simulink model "Allgemeine_Schematische"  (Simulink 7.7)
settings: Solver=ode45  StartTime=0.0  StopTime=12  MinStep=0.0001  RelTol=1e-3
undefined symbols (not defined in the file or in its folder): quad
libraries: simulink x4
settings Model: Creator=evgenov  LastModifiedBy=Alexey
settings DebuggingCC: FcnCallInpInsideContextMsg=Enable All

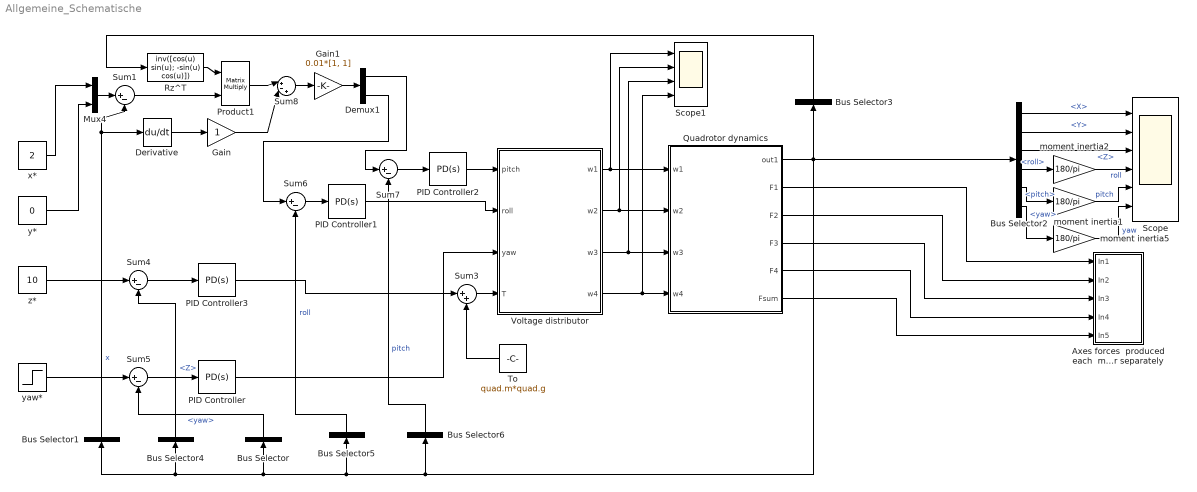
== system Allgemeine_Schematische ==
  Axes forces  produced each  motor separately : Subsystem
  Bus Selector : BusSelector  OutputSignals=yaw
  Bus Selector1 : BusSelector  OutputSignals=X,Y  OutputAsBus=on
  Bus Selector2 : BusSelector  OutputSignals=X,Y,Z,roll,pitch,yaw
  Bus Selector3 : BusSelector  OutputSignals=yaw  OutputAsBus=on
  Bus Selector4 : BusSelector  OutputSignals=Z
  Bus Selector5 : BusSelector  OutputSignals=roll  OutputAsBus=on
  Bus Selector6 : BusSelector  OutputSignals=pitch  OutputAsBus=on
  Demux1 : Demux  Outputs=2
  Derivative : Derivative
  Gain : Gain
  Gain1 : Gain  Gain=0.01*[1, 1]
  Mux4 : Mux  Inputs=2
  PID Controller : simulink/Continuous/PID Controller  SystemSampleTime=-1  Controller=PD  TimeDomain=Continuous-time  SampleTime=1  IntegratorMethod=Forward Euler  FilterMethod=Forward Euler  Form=Parallel  P=1  I=1  D=1  N=100  InitialConditionSource=internal  InitialConditionForIntegrator=0  InitialConditionForFilter=0  ExternalReset=none  LimitOutput=off  UpperSaturationLimit=inf  LowerSaturationLimit=-inf  LinearizeAsGain=off  AntiWindupMode=none  Kb=1  TrackingMode=off  Kt=1  PParamMin=[]  PParamMax=[]  IParamMin=[]  IParamMax=[]  DParamMin=[]  DParamMax=[]  NParamMin=[]  NParamMax=[]  KbParamMin=[]  KbParamMax=[]  KtParamMin=[]  KtParamMax=[]  POutMin=[]  POutMax=[]  IOutMin=[]  IOutMax=[]  DOutMin=[]  DOutMax=[]  NOutMin=[]  NOutMax=[]  KbOutMin=[]  KbOutMax=[]  KtOutMin=[]  KtOutMax=[]  IntegratorOutMin=[]  IntegratorOutMax=[]  FilterOutMin=[]  FilterOutMax=[]  SumOutMin=[]  SumOutMax=[]  SumI1OutMin=[]  SumI1OutMax=[]  SumI2OutMin=[]  SumI2OutMax=[]  SumI3OutMin=[]  SumI3OutMax=[]  SumDOutMin=[]  SumDOutMax=[]  SaturationOutMin=[]  SaturationOutMax=[]  IntegratorContinuousStateAttributes=''  IntegratorStateMustResolveToSignalObject=off  IntegratorRTWStateStorageClass=Auto  FilterContinuousStateAttributes=''  FilterStateMustResolveToSignalObject=off  FilterRTWStateStorageClass=Auto
  PID Controller1 : simulink/Continuous/PID Controller  SystemSampleTime=-1  Controller=PD  TimeDomain=Continuous-time  SampleTime=1  IntegratorMethod=Forward Euler  FilterMethod=Forward Euler  Form=Parallel  P=1  I=0  D=1  N=100  InitialConditionSource=internal  InitialConditionForIntegrator=0  InitialConditionForFilter=0  ExternalReset=none  LimitOutput=off  UpperSaturationLimit=inf  LowerSaturationLimit=-inf  LinearizeAsGain=off  AntiWindupMode=none  Kb=1  TrackingMode=off  Kt=1  PParamMin=[]  PParamMax=[]  IParamMin=[]  IParamMax=[]  DParamMin=[]  DParamMax=[]  NParamMin=[]  NParamMax=[]  KbParamMin=[]  KbParamMax=[]  KtParamMin=[]  KtParamMax=[]  POutMin=[]  POutMax=[]  IOutMin=[]  IOutMax=[]  DOutMin=[]  DOutMax=[]  NOutMin=[]  NOutMax=[]  KbOutMin=[]  KbOutMax=[]  KtOutMin=[]  KtOutMax=[]  IntegratorOutMin=[]  IntegratorOutMax=[]  FilterOutMin=[]  FilterOutMax=[]  SumOutMin=[]  SumOutMax=[]  SumI1OutMin=[]  SumI1OutMax=[]  SumI2OutMin=[]  SumI2OutMax=[]  SumI3OutMin=[]  SumI3OutMax=[]  SumDOutMin=[]  SumDOutMax=[]  SaturationOutMin=[]  SaturationOutMax=[]  IntegratorContinuousStateAttributes=''  IntegratorStateMustResolveToSignalObject=off  IntegratorRTWStateStorageClass=Auto  FilterContinuousStateAttributes=''  FilterStateMustResolveToSignalObject=off  FilterRTWStateStorageClass=Auto
  PID Controller2 : simulink/Continuous/PID Controller  SystemSampleTime=-1  Controller=PD  TimeDomain=Continuous-time  SampleTime=1  IntegratorMethod=Forward Euler  FilterMethod=Forward Euler  Form=Parallel  P=1  I=0  D=1  N=100  InitialConditionSource=internal  InitialConditionForIntegrator=0  InitialConditionForFilter=0  ExternalReset=none  LimitOutput=off  UpperSaturationLimit=inf  LowerSaturationLimit=-inf  LinearizeAsGain=off  AntiWindupMode=none  Kb=1  TrackingMode=off  Kt=1  PParamMin=[]  PParamMax=[]  IParamMin=[]  IParamMax=[]  DParamMin=[]  DParamMax=[]  NParamMin=[]  NParamMax=[]  KbParamMin=[]  KbParamMax=[]  KtParamMin=[]  KtParamMax=[]  POutMin=[]  POutMax=[]  IOutMin=[]  IOutMax=[]  DOutMin=[]  DOutMax=[]  NOutMin=[]  NOutMax=[]  KbOutMin=[]  KbOutMax=[]  KtOutMin=[]  KtOutMax=[]  IntegratorOutMin=[]  IntegratorOutMax=[]  FilterOutMin=[]  FilterOutMax=[]  SumOutMin=[]  SumOutMax=[]  SumI1OutMin=[]  SumI1OutMax=[]  SumI2OutMin=[]  SumI2OutMax=[]  SumI3OutMin=[]  SumI3OutMax=[]  SumDOutMin=[]  SumDOutMax=[]  SaturationOutMin=[]  SaturationOutMax=[]  IntegratorContinuousStateAttributes=''  IntegratorStateMustResolveToSignalObject=off  IntegratorRTWStateStorageClass=Auto  FilterContinuousStateAttributes=''  FilterStateMustResolveToSignalObject=off  FilterRTWStateStorageClass=Auto
  PID Controller3 : simulink/Continuous/PID Controller  SystemSampleTime=-1  Controller=PD  TimeDomain=Continuous-time  SampleTime=1  IntegratorMethod=Forward Euler  FilterMethod=Forward Euler  Form=Parallel  P=1  I=1  D=1.5  N=100  InitialConditionSource=internal  InitialConditionForIntegrator=0  InitialConditionForFilter=0  ExternalReset=none  LimitOutput=off  UpperSaturationLimit=inf  LowerSaturationLimit=-inf  LinearizeAsGain=off  AntiWindupMode=none  Kb=1  TrackingMode=off  Kt=1  PParamMin=[]  PParamMax=[]  IParamMin=[]  IParamMax=[]  DParamMin=[]  DParamMax=[]  NParamMin=[]  NParamMax=[]  KbParamMin=[]  KbParamMax=[]  KtParamMin=[]  KtParamMax=[]  POutMin=[]  POutMax=[]  IOutMin=[]  IOutMax=[]  DOutMin=[]  DOutMax=[]  NOutMin=[]  NOutMax=[]  KbOutMin=[]  KbOutMax=[]  KtOutMin=[]  KtOutMax=[]  IntegratorOutMin=[]  IntegratorOutMax=[]  FilterOutMin=[]  FilterOutMax=[]  SumOutMin=[]  SumOutMax=[]  SumI1OutMin=[]  SumI1OutMax=[]  SumI2OutMin=[]  SumI2OutMax=[]  SumI3OutMin=[]  SumI3OutMax=[]  SumDOutMin=[]  SumDOutMax=[]  SaturationOutMin=[]  SaturationOutMax=[]  IntegratorContinuousStateAttributes=''  IntegratorStateMustResolveToSignalObject=off  IntegratorRTWStateStorageClass=Auto  FilterContinuousStateAttributes=''  FilterStateMustResolveToSignalObject=off  FilterRTWStateStorageClass=Auto
  Product1 : Product  Multiplication=Matrix(*)  RndMeth=Zero
  Quadrotor dynamics : Subsystem
  Rz^T : MATLABFcn  MATLABFcn=inv([cos(u) sin(u); -sin(u) cos(u)])  OutputDimensions=[2 2]  Output1D=off
  Scope : Scope  NumInputPorts=6
      settings: TimeRange=2  YMin=-500~0~-1~-225~-30~-1000  YMax=100~800~1~-75~20~7000  SaveName=ScopeData2
  Scope1 : Scope  NumInputPorts=4
      settings: YMin=-5~-5~-5~-5  YMax=5~5~5~5
  Sum{1,4..7} (5 alike) : Sum  Inputs=|+-
  Sum3 : Sum  Inputs=|++
  Sum8 : Sum  Inputs=|+-+
  To : Constant  Value=quad.m*quad.g
  Voltage distributor : Subsystem
  moment inertia1 : Gain  Gain=180/pi
  moment inertia2 : Gain  Gain=180/pi
  moment inertia5 : Gain  Gain=180/pi
  x* : Constant  Value=2
  y* : Constant  Value=0
  yaw* : Step  Time=10  Before=0*pi/180  After=0*pi/180  SampleTime=0
  z* : Constant  Value=10
  wires:
  Quadrotor dynamics/1(out1) -> Bus Selector2/1, Bus Selector6/1, Bus Selector4/1, Bus Selector1/1, Bus Selector/1, Bus Selector5/1, Bus Selector3/1
  Bus Selector2/1 -> Scope/1  "<X>"
  Bus Selector2/2 -> Scope/2  "<Y>"
  Bus Selector2/3 -> Scope/3  "<Z>"
  Bus Selector2/4 -> moment inertia2/1  "<roll>"
  Bus Selector2/5 -> moment inertia1/1  "<pitch>"
  Bus Selector2/6 -> moment inertia5/1  "<yaw>"
  Quadrotor dynamics/2(F1) -> Axes forces  produced each  motor separately/1(In1)
  Quadrotor dynamics/3(F2) -> Axes forces  produced each  motor separately/2(In2)
  Quadrotor dynamics/4(F3) -> Axes forces  produced each  motor separately/3(In3)
  Quadrotor dynamics/5(F4) -> Axes forces  produced each  motor separately/4(In4)
  Quadrotor dynamics/6(Fsum) -> Axes forces  produced each  motor separately/5(In5)
  y*/1 -> Mux4/2
  Bus Selector/1 -> Sum5/2  "<yaw>"
  Bus Selector1/1 -> Sum1/2, Derivative/1  "x"
  Voltage distributor/1(w1) -> Quadrotor dynamics/1(w1), Scope1/1
  Voltage distributor/2(w2) -> Quadrotor dynamics/2(w2), Scope1/2
  Voltage distributor/3(w3) -> Quadrotor dynamics/3(w3), Scope1/3
  Voltage distributor/4(w4) -> Quadrotor dynamics/4(w4), Scope1/4
  moment inertia5/1 -> Scope/6  "yaw"
  moment inertia1/1 -> Scope/5  "pitch"
  moment inertia2/1 -> Scope/4  "roll"
  Bus Selector5/1 -> Sum6/2  "roll"
  Bus Selector4/1 -> Sum4/2  "<Z>"
  Bus Selector6/1 -> Sum7/2  "pitch"
  To/1 -> Sum3/2
  Sum4/1 -> PID Controller3/1
  yaw*/1 -> Sum5/1
  Sum5/1 -> PID Controller/1
  Sum6/1 -> PID Controller1/1
  Demux1/1 -> Sum7/1
  Sum7/1 -> PID Controller2/1
  PID Controller/1 -> Voltage distributor/3(yaw)
  Sum3/1 -> Voltage distributor/4(T)
  PID Controller1/1 -> Voltage distributor/2(roll)
  PID Controller2/1 -> Voltage distributor/1(pitch)
  PID Controller3/1 -> Sum3/1
  Rz^T/1 -> Product1/1
  Mux4/1 -> Sum1/1
  Bus Selector3/1 -> Rz^T/1
  Sum1/1 -> Product1/2
  Sum8/1 -> Gain1/1
  Product1/1 -> Sum8/1
  Derivative/1 -> Gain/1
  Gain/1 -> Sum8/2
  Gain1/1 -> Demux1/1
  Demux1/2 -> Sum6/1
  z*/1 -> Sum4/1
  x*/1 -> Mux4/1

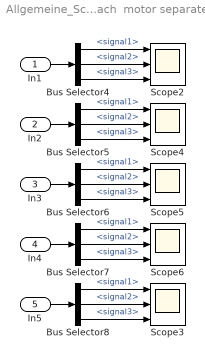
== system Allgemeine_Schematische/Axes forces  produced each  motor separately ==
  In1 : Inport
  In2 : Inport  Port=2
  In3 : Inport  Port=3
  In4 : Inport  Port=4
  In5 : Inport  Port=5
  Bus Selector{4..8} (5 alike) : BusSelector  OutputSignals=signal1,signal2,signal3
  Scope{2..6} (5 alike) : Scope  NumInputPorts=3
      Scope2 settings: TimeRange=20  YMin=0~0~0  YMax=800~800~800  SaveName=ScopeData3
      Scope3 settings: TimeRange=20  YMin=0~0~0  YMax=800~800~800
      Scope4 settings: TimeRange=20  YMin=0~0~0  YMax=800~800~800  SaveName=ScopeData4
      Scope5 settings: TimeRange=20  YMin=0~0~0  YMax=800~800~800  SaveName=ScopeData5
      Scope6 settings: TimeRange=20  YMin=0~0~0  YMax=800~800~800  SaveName=ScopeData6
  wires:
  Bus Selector4/1 -> Scope2/1  "<signal1>"
  Bus Selector4/2 -> Scope2/2  "<signal2>"
  Bus Selector4/3 -> Scope2/3  "<signal3>"
  Bus Selector5/1 -> Scope4/1  "<signal1>"
  Bus Selector5/2 -> Scope4/2  "<signal2>"
  Bus Selector5/3 -> Scope4/3  "<signal3>"
  Bus Selector6/1 -> Scope5/1  "<signal1>"
  Bus Selector6/2 -> Scope5/2  "<signal2>"
  Bus Selector6/3 -> Scope5/3  "<signal3>"
  Bus Selector7/1 -> Scope6/1  "<signal1>"
  Bus Selector7/2 -> Scope6/2  "<signal2>"
  Bus Selector7/3 -> Scope6/3  "<signal3>"
  Bus Selector8/1 -> Scope3/1  "<signal1>"
  Bus Selector8/2 -> Scope3/2  "<signal2>"
  Bus Selector8/3 -> Scope3/3  "<signal3>"
  In1/1 -> Bus Selector4/1
  In2/1 -> Bus Selector5/1
  In3/1 -> Bus Selector6/1
  In4/1 -> Bus Selector7/1
  In5/1 -> Bus Selector8/1

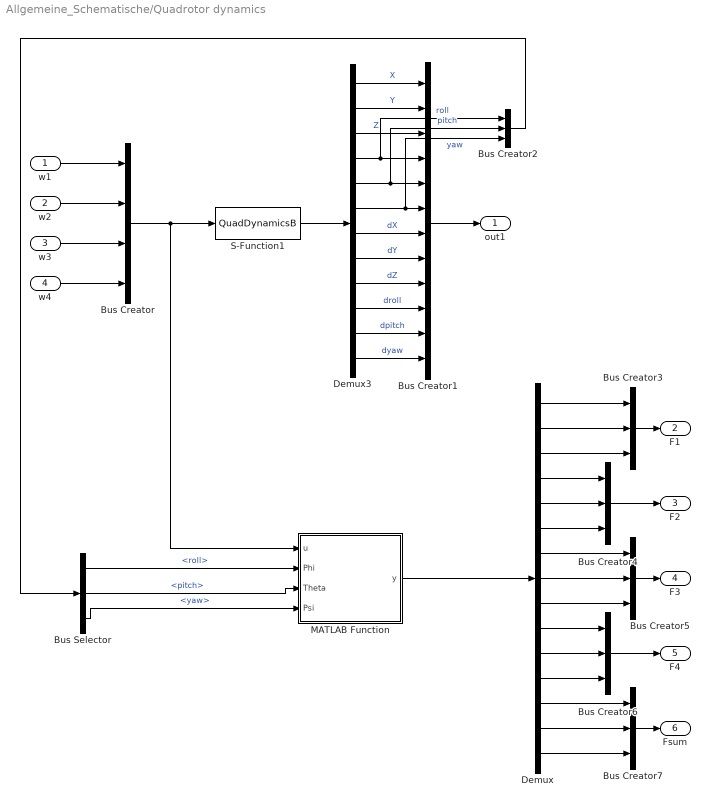
== system Allgemeine_Schematische/Quadrotor dynamics ==
  w1 : Inport
  w2 : Inport  Port=2
  w3 : Inport  Port=3
  w4 : Inport  Port=4
  Bus Creator : BusCreator
  Bus Creator1 : BusCreator  Inputs=12
  Bus Creator{2..7} (6 alike) : BusCreator  Inputs=3
  Bus Selector : BusSelector  OutputSignals=roll,pitch,yaw
  Demux : Demux  Outputs=15
  Demux3 : Demux  Outputs=12
  MATLAB Function : Stateflow chart  TreatAsAtomicUnit=on
  S-Function1 : S-Function  FunctionName=QuadDynamicsB  Parameters=quad  EnableBusSupport=off
  out1 : Outport
  F1 : Outport  Port=2
  F2 : Outport  Port=3
  F3 : Outport  Port=4
  F4 : Outport  Port=5
  Fsum : Outport  Port=6
  wires:
  w1/1 -> Bus Creator/1
  w2/1 -> Bus Creator/2
  w3/1 -> Bus Creator/3
  w4/1 -> Bus Creator/4
  Bus Creator1/1 -> out1/1
  Bus Creator/1 -> S-Function1/1, MATLAB Function/1(u)
  Demux3/1 -> Bus Creator1/1  "X"
  Demux3/2 -> Bus Creator1/2  "Y"
  Demux3/3 -> Bus Creator1/3  "Z"
  Demux3/4 -> Bus Creator2/1, Bus Creator1/4  "roll"
  Demux3/5 -> Bus Creator1/5, Bus Creator2/2  "pitch"
  Demux3/6 -> Bus Creator1/6, Bus Creator2/3  "yaw"
  Demux3/7 -> Bus Creator1/7  "dX"
  Demux3/8 -> Bus Creator1/8  "dY"
  Demux3/9 -> Bus Creator1/9  "dZ"
  Demux3/10 -> Bus Creator1/10  "droll"
  Demux3/11 -> Bus Creator1/11  "dpitch"
  Demux3/12 -> Bus Creator1/12  "dyaw"
  S-Function1/1 -> Demux3/1
  MATLAB Function/1(y) -> Demux/1
  Bus Creator2/1 -> Bus Selector/1
  Bus Selector/1 -> MATLAB Function/2(Phi)  "<roll>"
  Bus Selector/2 -> MATLAB Function/3(Theta)  "<pitch>"
  Bus Selector/3 -> MATLAB Function/4(Psi)  "<yaw>"
  Demux/1 -> Bus Creator3/1
  Demux/2 -> Bus Creator3/2
  Demux/3 -> Bus Creator3/3
  Demux/4 -> Bus Creator4/1
  Demux/5 -> Bus Creator4/2
  Demux/6 -> Bus Creator4/3
  Demux/7 -> Bus Creator5/1
  Demux/8 -> Bus Creator5/2
  Demux/9 -> Bus Creator5/3
  Demux/10 -> Bus Creator6/1
  Demux/11 -> Bus Creator6/2
  Demux/12 -> Bus Creator6/3
  Demux/13 -> Bus Creator7/1
  Demux/14 -> Bus Creator7/2
  Demux/15 -> Bus Creator7/3
  Bus Creator3/1 -> F1/1
  Bus Creator4/1 -> F2/1
  Bus Creator5/1 -> F3/1
  Bus Creator6/1 -> F4/1
  Bus Creator7/1 -> Fsum/1

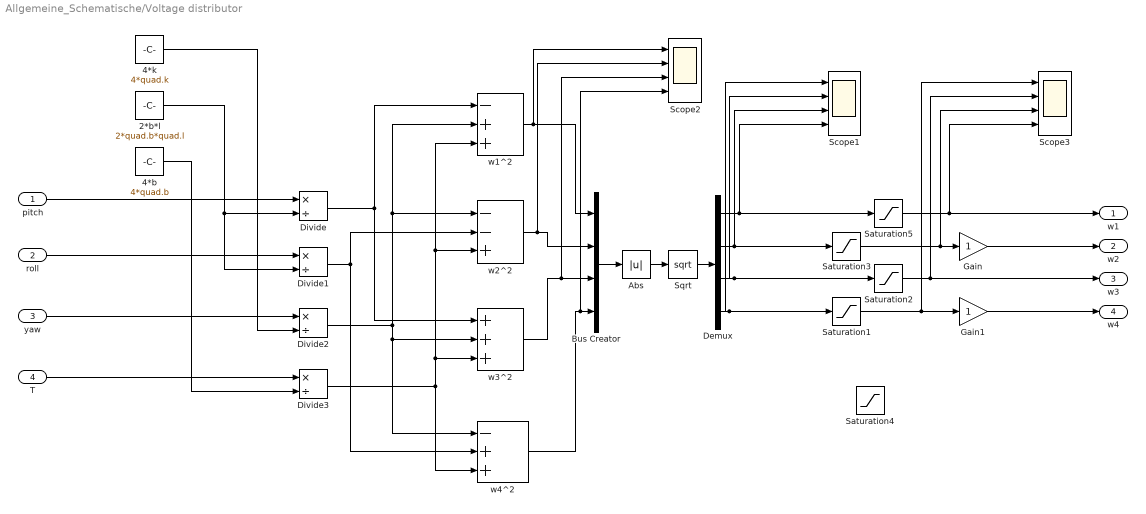
== system Allgemeine_Schematische/Voltage distributor ==
  pitch : Inport
  roll : Inport  Port=2
  yaw : Inport  Port=3
  T : Inport  Port=4
  2*b*l : Constant  Value=2*quad.b*quad.l
  4*b : Constant  Value=4*quad.b
  4*k : Constant  Value=4*quad.k
  Abs : Abs  ZeroCross=off
  Bus Creator : BusCreator
  Demux : Demux
  Divide{,1..3} (4 alike) : Product  Inputs=*/
  Gain : Gain
  Gain1 : Gain
  Saturation{1..5} (5 alike) : Saturate  UpperLimit=1000  LowerLimit=500  ZeroCross=off
  Scope1 : Scope  NumInputPorts=4
      settings: YMin=-5~-5~-5~-5  YMax=5~5~5~5  SaveName=ScopeData8
  Scope2 : Scope  NumInputPorts=4
      settings: YMin=-1.5e+007~-2.5e+006~-1.5e+007~-2.5e+006  YMax=2.5e+006~1.25e+007~2.5e+006~1.25e+007  SaveName=ScopeData9
  Scope3 : Scope  NumInputPorts=4
      settings: YMin=-5~-5~-5~-5  YMax=5~5~5~5  SaveName=ScopeData7
  Sqrt : Sqrt  SaturateOnIntegerOverflow=on
  w1^2 : Sum  Inputs=-++
  w2^2 : Sum  Inputs=--+
  w3^2 : Sum  Inputs=+++
  w4^2 : Sum  Inputs=-++
  w1 : Outport
  w2 : Outport  Port=2
  w3 : Outport  Port=3
  w4 : Outport  Port=4
  wires:
  4*k/1 -> Divide2/2
  Divide1/1 -> w4^2/2, w2^2/2
  Divide2/1 -> w3^2/2, w4^2/1, w2^2/1, w1^2/2
  Divide/1 -> w3^2/1, w1^2/1
  4*b/1 -> Divide3/2
  yaw/1 -> Divide2/1
  2*b*l/1 -> Divide/2, Divide1/2
  roll/1 -> Divide1/1
  pitch/1 -> Divide/1
  Bus Creator/1 -> Abs/1
  Sqrt/1 -> Demux/1
  w1^2/1 -> Bus Creator/1, Scope2/1
  w2^2/1 -> Bus Creator/2, Scope2/2
  w3^2/1 -> Bus Creator/3, Scope2/3
  w4^2/1 -> Bus Creator/4, Scope2/4
  Demux/1 -> Scope1/4, Saturation5/1
  Demux/2 -> Scope1/3, Saturation3/1
  Demux/3 -> Scope1/2, Saturation2/1
  Demux/4 -> Scope1/1, Saturation1/1
  Divide3/1 -> w2^2/3, w1^2/3, w3^2/3, w4^2/3
  Abs/1 -> Sqrt/1
  Gain/1 -> w2/1
  Gain1/1 -> w4/1
  T/1 -> Divide3/1
  Saturation5/1 -> w1/1, Scope3/4
  Saturation3/1 -> Gain/1, Scope3/3
  Saturation2/1 -> w3/1, Scope3/2
  Saturation1/1 -> Gain1/1, Scope3/1

== matlab function Quadrotor dynamics/MATLAB Function ==
  data: u input double; y output double; Phi input double; Theta input double; Psi input double
function y = fcn(u,Phi,Theta,Psi)
%#codegen
T=zeros(12,1);
b=9.7575e-6;
w2=([u(1);u(2);u(3);u(4)]).^2;

Rx=[1 0 0; 0 cos(Phi) -sin(Phi); 0 sin(Phi) cos(Phi)];
Ry=[cos(Theta) 0 sin(Theta); 0 1 0; -sin(Theta) 0 cos(Theta)];
Rz=[cos(Psi) -sin(Psi) 0; sin(Psi) cos(Psi) 0; 0 0 1];
R=Rx*Ry*Rz;
k=0;
for i=1:4
        f=R*[0;0;b*w2(i)];
        for j=1:3
           k=k+1;
           T(k)=f(j);
        end;
end;

F=R*[0;0;b*sum(w2)];
y = [T; F];
